simulink model "Verification_simulink_restored_from_autosave"  (R2023a)
settings: Solver=ode15s  StartTime=0.0  StopTime=13  MaxStep=0.001  RelTol=1e-3
values from neighbouring files (symbols this model uses):
  A = [0, 1, 0;K/I, -b_p/I, b_w/I;-K/I, b_p/I, -b_w*I_r]    [LQR.m]    (also in model_verif.m = [0, 1, 0, 0;-K/I, -b_p/I, 0, -b_w/I;0, 0, 0, 1;K/I, b_p/I, 0)
  B = [0;-K_m/I;I_r*K_m]    [LQR.m]    (also in model_verif.m = [0, 0;-K_m/I, 1/I;0, 0;I_r*K_m, -1/I])
  b_p = 0.0314    [CascadePID.m]    (also in LQR.m; model_verif.m = 0.0114)
  b_w = 1/(T*I_r)    (= 0.000346638655462)    [CascadePID.m]    (also in LQR.m; model_verif.m = 0.000315333070556)
  C = tf(num_C,denom_C)    [CascadePID.m]    (also in LQR.m = [1 0 0;0 1 0;0 0 1]; model_verif.m = [1 0 0 0;0 1 0 0;0 0 1 0;0 0 0 1])
  I = 0.011    [CascadePID.m]    (also in LQR.m; model_verif.m = 0.012)
  I_r = (I+I_w)/(I*I_w)    (= 424.242424242)    [CascadePID.m]    (also in LQR.m; model_verif.m = 416.666666667)
  K = 0.597    [CascadePID.m]    (also in Identification_TF.m = X(1); LQR.m; cost_TF.m = ',num2str(K),'; model_verif.m)
  K_m = G*b_w    (= 2.59112394958)    [CascadePID.m]    (also in LQR.m; model_verif.m = 2.3571147024)
  x0 = [20; 0; 0; 0]    [LQR.m]
undefined symbols (not defined in the file or in its folder): DiscIntNeverNeededParam
libraries: slpidlib x3, simulink x1
settings Model: Creator=claraneuburger  LastModifiedBy=claraneuburger

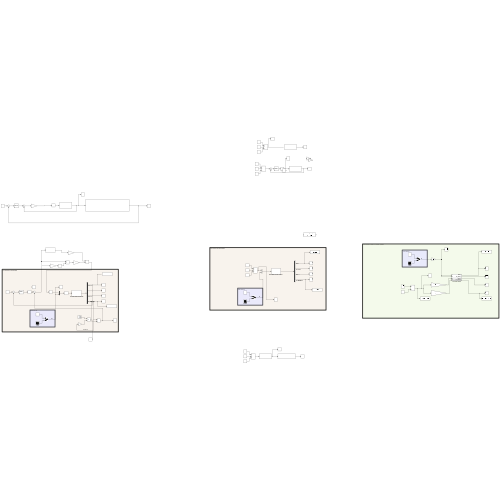
[thumbnail: Simulink's stored preview of the top-level diagram]
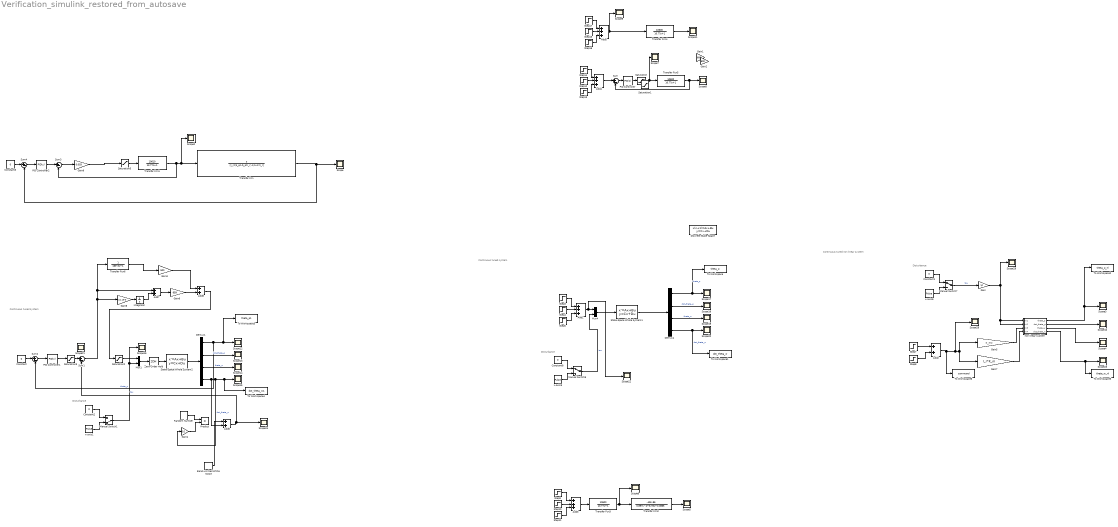
== system Verification_simulink_restored_from_autosave ==
  note: Disturbance
  note: Continuous tuned system
  note: Disturbance
  note: Continuous tuned non linear system
  note: Continuous tuned system
  note: Disturbance
  Add{1,3..5} (4 alike) : Sum  Inputs=+++
  Add{2,6..8} (4 alike) : Sum
  Band-Limited White Noise : simulink/Sources/Band-Limited White Noise  Cov=[0.05]  Ts=0.01  seed=[23341]
  Constant{,1..3,8} (5 alike) : Constant  Value=0
  Demux1 : Demux
  Demux4 : Demux
  Discrete State-Space : DiscreteStateSpace  A=A  B=B  C=C  D=[0,0;0,0;0,0;0,0]  InitialCondition=x0  SampleTime=0.01
  Gain : Gain  Gain=1/I
  Gain1 : Gain  Gain=600
  Gain2 : Gain  Gain=600
  Gain3 : Gain  Gain=500
  Gain4 : Gain  Gain=0.1
  Gain5 : Gain  Gain=K_m/I
  Gain6 : Gain  Gain=659
  Gain7 : Gain  Gain=I_r*K_m
  Gain8 : Gain  Gain=22.1e-3
  Gain9 : Gain  Gain=0.003
  Integrator : Integrator
  Manual Switch1 : ManualSwitch  CurrentSetting=0
  Manual Switch6 : ManualSwitch
  Manual Switch7 : ManualSwitch
  Mux1 : Mux  Inputs=2
  Mux4 : Mux  Inputs=2
  PID Controller : slpidlib/PID Controller  Controller=PID  Form=Parallel  TimeDomain=Continuous-time  UseExternalTs=off  SampleTime=-1  IntegratorMethod=Forward Euler  FilterMethod=Forward Euler  ControllerParametersSource=internal  P=0.002  I=0  UseKiTs=off  D=0  N=0  UseFilter=on  TunerSelectOption=Transfer Function Based (PID Tuner App)  InitialConditionSource=internal  InitialConditionForIntegrator=0  InitialConditionForFilter=0  DifferentiatorICPrevScaledInput=0  ExternalReset=none  TrackingMode=off  Kt=1  LimitOutput=off  SatLimitsSource=internal  UpperSaturationLimit=inf  LowerSaturationLimit=-inf  LinearizeAsGain=on  AntiWindupMode=none  Kb=1  LimitIntegrator=off  UpperIntegratorSaturationLimit=inf  LowerIntegratorSaturationLimit=-inf  POutMin=[]  POutMax=[]  IOutMin=[]  IOutMax=[]  DOutMin=[]  DOutMax=[]  NOutMin=[]  NOutMax=[]  SumOutMin=[]  SumOutMax=[]  SaturationOutMin=[]  SaturationOutMax=[]  PParamMin=[]  PParamMax=[]  IParamMin=[]  IParamMax=[]  DParamMin=[]  DParamMax=[]  NParamMin=[]  NParamMax=[]  KbParamMin=[]  KbParamMax=[]  KtParamMin=[]  KtParamMax=[]  KbOutMin=[]  KbOutMax=[]  KtOutMin=[]  KtOutMax=[]  IntegratorOutMin=[]  IntegratorOutMax=[]  FilterOutMin=[]  FilterOutMax=[]  SumI1OutMin=[]  SumI1OutMax=[]  SumI2OutMin=[]  SumI2OutMax=[]  SumI3OutMin=[]  SumI3OutMax=[]  SumI4OutMin=[]  SumI4OutMax=[]  SumDOutMin=[]  SumDOutMax=[]  DifferentiatorOutMin=[]  DifferentiatorOutMax=[]  FilterDiffOutCoefMin=[]  FilterDiffOutCoefMax=[]  ReciprocalOutMin=[]  ReciprocalOutMax=[]  SumDenOutMin=[]  SumDenOutMax=[]  SumNumOutMin=[]  SumNumOutMax=[]  DivideOutMin=[]  DivideOutMax=[]  UdiffTsProdOutMin=[]  UdiffTsProdOutMax=[]  NTsProdOutMin=[]  NTsProdOutMax=[]  UintegralTsProdOutMin=[]  UintegralTsProdOutMax=[]  UngainTsProdOutMin=[]  UngainTsProdOutMax=[]  ClampingZeroOutDataTypeStr=Inherit: Inherit via back propagation  ClampingZeroOutMin=[]  ClampingZeroOutMax=[]  FilterDenConstantOutDataTypeStr=Inherit: Inherit via back propagation  FilterDenConstantOutMin=[]  FilterDenConstantOutMax=[]  PCopyOutDataTypeStr=Inherit: Inherit via back propagation  PCopyOutMin=[]  PCopyOutMax=[]  NCopyOutDataTypeStr=Inherit: Inherit via back propagation  NCopyOutMin=[]  NCopyOutMax=[]  IntegratorContinuousStateAttributes=''  IntegratorStateMustResolveToSignalObject=off  IntegratorRTWStateStorageClass=Auto  FilterContinuousStateAttributes=''  FilterStateMustResolveToSignalObject=off  FilterRTWStateStorageClass=Auto  ParallelPVariant=InternalParameters  IdealPVariant=Disabled  IVariant=InternalParameters  DVariant=InternalParameters  IntegratorVariant=Continuous  SatVariant=Disabled  AWVariant=Passthrough  PCopyVariant=Disabled  TRVariant=Disabled  FdbkBlocksVariant=Forward  IdealPFdbkVariant=Disabled  SatFdbkVariant=Disabled  DerivativeFilterVariant=ContFilter  NVariant=InternalParameters  NCopyVariant=Disabled  FilterICVariant=InternalICsFilter  IntegratorICVariant=InternalICs  ExternalResetVariant=Disabled  TRSumVariant=Passthrough  SumFdbkVariant=Disabled  SumVariant=Sum_PID  TsampFilterVariant=InternalTs  TsampNgainVariant=Passthrough  TsampIntegralVariant=Disabled_SignalSpec  ExternalSaturationOutDataTypeStr=Inherit: Same as second input
  PID Controller1 : slpidlib/PID Controller  Controller=PID  Form=Parallel  TimeDomain=Discrete-time  UseExternalTs=off  SampleTime=0.01  IntegratorMethod=Forward Euler  FilterMethod=Forward Euler  ControllerParametersSource=internal  P=-3941.34808580242  I=-19558.7721008802  UseKiTs=off  D=-188.491586506074  N=193.809190718502  UseFilter=on  TunerSelectOption=Transfer Function Based (PID Tuner App)  InitialConditionSource=internal  InitialConditionForIntegrator=0  InitialConditionForFilter=0  DifferentiatorICPrevScaledInput=0  ExternalReset=none  TrackingMode=off  Kt=1  LimitOutput=off  SatLimitsSource=internal  UpperSaturationLimit=inf  LowerSaturationLimit=-inf  LinearizeAsGain=on  AntiWindupMode=none  Kb=1  LimitIntegrator=off  UpperIntegratorSaturationLimit=inf  LowerIntegratorSaturationLimit=-inf  POutMin=[]  POutMax=[]  IOutMin=[]  IOutMax=[]  DOutMin=[]  DOutMax=[]  NOutMin=[]  NOutMax=[]  SumOutMin=[]  SumOutMax=[]  SaturationOutMin=[]  SaturationOutMax=[]  PParamMin=[]  PParamMax=[]  IParamMin=[]  IParamMax=[]  DParamMin=[]  DParamMax=[]  NParamMin=[]  NParamMax=[]  KbParamMin=[]  KbParamMax=[]  KtParamMin=[]  KtParamMax=[]  KbOutMin=[]  KbOutMax=[]  KtOutMin=[]  KtOutMax=[]  IntegratorOutMin=[]  IntegratorOutMax=[]  FilterOutMin=[]  FilterOutMax=[]  SumI1OutMin=[]  SumI1OutMax=[]  SumI2OutMin=[]  SumI2OutMax=[]  SumI3OutMin=[]  SumI3OutMax=[]  SumI4OutMin=[]  SumI4OutMax=[]  SumDOutMin=[]  SumDOutMax=[]  DifferentiatorOutMin=[]  DifferentiatorOutMax=[]  FilterDiffOutCoefMin=[]  FilterDiffOutCoefMax=[]  ReciprocalOutMin=[]  ReciprocalOutMax=[]  SumDenOutMin=[]  SumDenOutMax=[]  SumNumOutMin=[]  SumNumOutMax=[]  DivideOutMin=[]  DivideOutMax=[]  UdiffTsProdOutMin=[]  UdiffTsProdOutMax=[]  NTsProdOutMin=[]  NTsProdOutMax=[]  UintegralTsProdOutMin=[]  UintegralTsProdOutMax=[]  UngainTsProdOutMin=[]  UngainTsProdOutMax=[]  ClampingZeroOutDataTypeStr=Inherit: Inherit via back propagation  ClampingZeroOutMin=[]  ClampingZeroOutMax=[]  FilterDenConstantOutDataTypeStr=Inherit: Inherit via back propagation  FilterDenConstantOutMin=[]  FilterDenConstantOutMax=[]  PCopyOutDataTypeStr=Inherit: Inherit via back propagation  PCopyOutMin=[]  PCopyOutMax=[]  NCopyOutDataTypeStr=Inherit: Inherit via back propagation  NCopyOutMin=[]  NCopyOutMax=[]  IntegratorContinuousStateAttributes=''  IntegratorStateMustResolveToSignalObject=off  IntegratorRTWStateStorageClass=Auto  FilterContinuousStateAttributes=''  FilterStateMustResolveToSignalObject=off  FilterRTWStateStorageClass=Auto  ParallelPVariant=InternalParameters  IdealPVariant=Disabled  IVariant=InternalParameters  DVariant=InternalParameters  IntegratorVariant=Discrete  SatVariant=Disabled  AWVariant=Passthrough  PCopyVariant=Disabled  TRVariant=Disabled  FdbkBlocksVariant=Forward  IdealPFdbkVariant=Disabled  SatFdbkVariant=Disabled  DerivativeFilterVariant=ForwardEulerFilter  NVariant=InternalParameters  NCopyVariant=Disabled  FilterICVariant=InternalICsFilter  IntegratorICVariant=InternalICs  ExternalResetVariant=Disabled  TRSumVariant=Passthrough  SumFdbkVariant=Disabled  SumVariant=Sum_PID  TsampFilterVariant=InternalTs  TsampNgainVariant=Passthrough  TsampIntegralVariant=Disabled_SignalSpec  ExternalSaturationOutDataTypeStr=Inherit: Same as second input
  PID Controller2 : slpidlib/PID Controller  Controller=PID  Form=Parallel  TimeDomain=Discrete-time  UseExternalTs=off  SampleTime=0.01  IntegratorMethod=Forward Euler  FilterMethod=Forward Euler  ControllerParametersSource=internal  P=130515.507313953  I=39331.7681676177  UseKiTs=off  D=-1038.52898929221  N=77.1061222235788  UseFilter=on  TunerSelectOption=Transfer Function Based (PID Tuner App)  InitialConditionSource=internal  InitialConditionForIntegrator=0  InitialConditionForFilter=0  DifferentiatorICPrevScaledInput=0  ExternalReset=none  TrackingMode=off  Kt=1  LimitOutput=off  SatLimitsSource=internal  UpperSaturationLimit=inf  LowerSaturationLimit=-inf  LinearizeAsGain=on  AntiWindupMode=none  Kb=1  LimitIntegrator=off  UpperIntegratorSaturationLimit=inf  LowerIntegratorSaturationLimit=-inf  POutMin=[]  POutMax=[]  IOutMin=[]  IOutMax=[]  DOutMin=[]  DOutMax=[]  NOutMin=[]  NOutMax=[]  SumOutMin=[]  SumOutMax=[]  SaturationOutMin=[]  SaturationOutMax=[]  PParamMin=[]  PParamMax=[]  IParamMin=[]  IParamMax=[]  DParamMin=[]  DParamMax=[]  NParamMin=[]  NParamMax=[]  KbParamMin=[]  KbParamMax=[]  KtParamMin=[]  KtParamMax=[]  KbOutMin=[]  KbOutMax=[]  KtOutMin=[]  KtOutMax=[]  IntegratorOutMin=[]  IntegratorOutMax=[]  FilterOutMin=[]  FilterOutMax=[]  SumI1OutMin=[]  SumI1OutMax=[]  SumI2OutMin=[]  SumI2OutMax=[]  SumI3OutMin=[]  SumI3OutMax=[]  SumI4OutMin=[]  SumI4OutMax=[]  SumDOutMin=[]  SumDOutMax=[]  DifferentiatorOutMin=[]  DifferentiatorOutMax=[]  FilterDiffOutCoefMin=[]  FilterDiffOutCoefMax=[]  ReciprocalOutMin=[]  ReciprocalOutMax=[]  SumDenOutMin=[]  SumDenOutMax=[]  SumNumOutMin=[]  SumNumOutMax=[]  DivideOutMin=[]  DivideOutMax=[]  UdiffTsProdOutMin=[]  UdiffTsProdOutMax=[]  NTsProdOutMin=[]  NTsProdOutMax=[]  UintegralTsProdOutMin=[]  UintegralTsProdOutMax=[]  UngainTsProdOutMin=[]  UngainTsProdOutMax=[]  ClampingZeroOutDataTypeStr=Inherit: Inherit via back propagation  ClampingZeroOutMin=[]  ClampingZeroOutMax=[]  FilterDenConstantOutDataTypeStr=Inherit: Inherit via back propagation  FilterDenConstantOutMin=[]  FilterDenConstantOutMax=[]  PCopyOutDataTypeStr=Inherit: Inherit via back propagation  PCopyOutMin=[]  PCopyOutMax=[]  NCopyOutDataTypeStr=Inherit: Inherit via back propagation  NCopyOutMin=[]  NCopyOutMax=[]  IntegratorContinuousStateAttributes=''  IntegratorStateMustResolveToSignalObject=off  IntegratorRTWStateStorageClass=Auto  FilterContinuousStateAttributes=''  FilterStateMustResolveToSignalObject=off  FilterRTWStateStorageClass=Auto  ParallelPVariant=InternalParameters  IdealPVariant=Disabled  IVariant=InternalParameters  DVariant=InternalParameters  IntegratorVariant=Discrete  SatVariant=Disabled  AWVariant=Passthrough  PCopyVariant=Disabled  TRVariant=Disabled  FdbkBlocksVariant=Forward  IdealPFdbkVariant=Disabled  SatFdbkVariant=Disabled  DerivativeFilterVariant=ForwardEulerFilter  NVariant=InternalParameters  NCopyVariant=Disabled  FilterICVariant=InternalICsFilter  IntegratorICVariant=InternalICs  ExternalResetVariant=Disabled  TRSumVariant=Passthrough  SumFdbkVariant=Disabled  SumVariant=Sum_PID  TsampFilterVariant=InternalTs  TsampNgainVariant=Passthrough  TsampIntegralVariant=Disabled_SignalSpec  ExternalSaturationOutDataTypeStr=Inherit: Same as second input
  Product : Product
  Random Number : RandomNumber  SampleTime=0.001
  Saturation{,1..2,5} (4 alike) : Saturate  UpperLimit=2.33  LowerLimit=-2.33
  Saturation3 : Saturate  UpperLimit=10  LowerLimit=-10
  Scope{,2..24,28..29} (26 alike) : Scope
  State-Space Whole System1 : StateSpace  A=A  B=B  C=C  D=[0,0;0,0;0,0;0,0]  InitialCondition=x0
  State-Space Whole System2 : StateSpace  A=A  B=B  C=C  D=[0,0;0,0;0,0;0,0]  InitialCondition=x0
  Step10 : Step  Time=15  After=0.31772  SampleTime=0
  Step11 : Step  Time=19  After=-0.31772  SampleTime=0
  Step12 : Step  Time=15  After=1000  SampleTime=0
  Step13 : Step  Time=19  After=-1000  SampleTime=0
  Step{3,7,9,14,17} (5 alike) : Step  Time=0  After=0  SampleTime=0
  Step15 : Step  Time=15  After=0.31772  SampleTime=0
  Step16 : Step  Time=19  After=-0.31772  SampleTime=0
  Step4 : Step  Time=15  After=0.74  SampleTime=0
  Step5 : Step  Time=16  After=-0.74  SampleTime=0
  Step8 : Step  Before=1  After=0  SampleTime=0
  Sum{,1..4} (5 alike) : Sum  Inputs=|+-
  To Workspace : ToWorkspace  VariableName=theta_p  SaveFormat=Timeseries  SampleTime=-1
  To Workspace1 : ToWorkspace  VariableName=dot_theta_w  SaveFormat=Timeseries  SampleTime=-1
  To Workspace2 : ToWorkspace  VariableName=theta_p_nl  SaveFormat=Timeseries  SampleTime=-1
  To Workspace3 : ToWorkspace  VariableName=theta_p1  SaveFormat=Timeseries  SampleTime=-1
  To Workspace4 : ToWorkspace  VariableName=dot_theta_w1  SaveFormat=Timeseries  SampleTime=-1
  To Workspace5 : ToWorkspace  VariableName=theta_w_nl  SaveFormat=Timeseries  SampleTime=-1
  To Workspace6 : ToWorkspace  VariableName=command  SaveFormat=Timeseries  SampleTime=-1
  Transfer Fcn : TransferFcn  Numerator=[1 0]  Denominator=[I_r/I;b_p/I-b_p*I_r;-K/I+K*I_r]
  Transfer Fcn1 : TransferFcn  Numerator=[10610]  Denominator=[13.77 1]
  Transfer Fcn2 : TransferFcn  Numerator=[-49 -86]  Denominator=[0.897 8.78 0.0865]
  Transfer Fcn3 : TransferFcn  Numerator=[10600]  Denominator=[10.77 1]
  Transfer Fcn4 : TransferFcn  Numerator=[10600]  Denominator=[10.77 1]
  Transfer Fcn5 : TransferFcn  Numerator=[10600]  Denominator=[10.77 1]
  Transfer Fcn6 : TransferFcn  Denominator=[16e-3 1]
  Zero-Order Hold : ZeroOrderHold  SampleTime=0.01
  non linear system : Subsystem
  x-axis1 : DiscretePulseGenerator  PulseType=Time based  Amplitude=2  Period=17  PulseWidth=0.01  PhaseDelay=1
  x-axis5 : DiscretePulseGenerator  PulseType=Time based  Amplitude=2  Period=17  PulseWidth=0.01  PhaseDelay=1
  x-axis6 : DiscretePulseGenerator  PulseType=Time based  Amplitude=2  Period=1  PulseWidth=0.5  PhaseDelay=1
  wires:
  Transfer Fcn1/1 -> Sum3/2, Transfer Fcn/1, Scope2/1
  Transfer Fcn/1 -> Sum4/2, Scope/1
  Demux4/3 -> Scope19/1  "theta_w"
  Demux4/1 -> To Workspace/1, Scope17/1  "theta_p"
  Manual Switch6/1 -> Mux4/2  "tau"
  Demux4/4 -> To Workspace1/1, Scope20/1  "dot_theta_w"
  x-axis5/1 -> Manual Switch6/2
  Demux4/2 -> Scope18/1  "dot_theta_p"
  Constant8/1 -> Manual Switch6/1
  Step5/1 -> Add1/3
  Step4/1 -> Add1/2
  Step3/1 -> Add1/1
  Constant1/1 -> Manual Switch7/1
  Gain5/1 -> non linear system/3(In3)
  Manual Switch7/1 -> Gain/1  "tau"
  x-axis6/1 -> Manual Switch7/2
  Gain7/1 -> non linear system/4(In4)
  non linear system/1(theta_p) -> To Workspace2/1, Scope3/1
  Gain/1 -> Scope29/1, non linear system/2(In2), non linear system/1(In1)
  non linear system/2(dot_theta_p) -> Scope10/1
  non linear system/3(theta_w) -> Scope4/1
  non linear system/4(dot_theta_w) -> To Workspace5/1, Scope23/1
  Add2/1 -> To Workspace6/1, Scope28/1, Gain7/1, Gain5/1
  Step8/1 -> Add2/2
  Mux4/1 -> State-Space Whole System1/1
  State-Space Whole System1/1 -> Demux4/1
  Add1/1 -> Scope22/1, Mux4/1
  Step7/1 -> Add2/1
  Step11/1 -> Add3/3
  Step10/1 -> Add3/2
  Step9/1 -> Add3/1
  Transfer Fcn3/1 -> Scope6/1, Transfer Fcn2/1
  Add3/1 -> Transfer Fcn3/1
  Transfer Fcn2/1 -> Scope5/1
  Step12/1 -> Add4/2
  Transfer Fcn5/1 -> Sum/2, Scope8/1
  Step14/1 -> Add4/1
  Step13/1 -> Add4/3
  Add4/1 -> Sum/1
  Step15/1 -> Add5/2
  Step16/1 -> Add5/3
  Add5/1 -> Transfer Fcn4/1, Scope9/1
  Transfer Fcn4/1 -> Scope11/1
  Step17/1 -> Add5/1
  Sum/1 -> PID Controller/1
  PID Controller/1 -> Saturation/1
  Saturation/1 -> Scope7/1, Transfer Fcn5/1
  State-Space Whole System2/1 -> Demux1/1
  Demux1/3 -> Scope14/1  "theta_w"
  x-axis1/1 -> Manual Switch1/2
  Constant2/1 -> Manual Switch1/1
  Demux1/1 -> To Workspace3/1, Scope12/1, Sum2/2  "theta_p"
  Demux1/4 -> Gain4/1, To Workspace4/1, Scope15/1, Add6/2  "dot_theta_w"
  Manual Switch1/1 -> Scope16/1, Mux1/2  "tau"
  Demux1/2 -> Scope13/1  "dot_theta_p"
  Mux1/1 -> Zero-Order Hold/1
  Saturation2/1 -> Mux1/1
  Sum2/1 -> PID Controller1/1
  Constant/1 -> Sum2/1
  Zero-Order Hold/1 -> State-Space Whole System2/1
  Random Number/1 -> Product/1
  Gain4/1 -> Product/2
  Band-Limited White Noise/1 -> Add6/1
  PID Controller1/1 -> Saturation3/1
  Add6/1 -> Sum1/2, Scope24/1
  Saturation3/1 -> Sum1/1
  Add8/1 -> Saturation2/1
  Sum1/1 -> Gain8/1, Transfer Fcn6/1, Add7/1
  Gain8/1 -> Integrator/1
  Integrator/1 -> Add7/2
  Gain6/1 -> Add8/2
  Add7/1 -> Gain6/1
  Transfer Fcn6/1 -> Gain3/1
  Gain3/1 -> Add8/1
  Sum4/1 -> PID Controller2/1
  Constant3/1 -> Sum4/1
  PID Controller2/1 -> Sum3/1
  Saturation5/1 -> Transfer Fcn1/1
  Sum3/1 -> Gain9/1
  Gain9/1 -> Saturation5/1

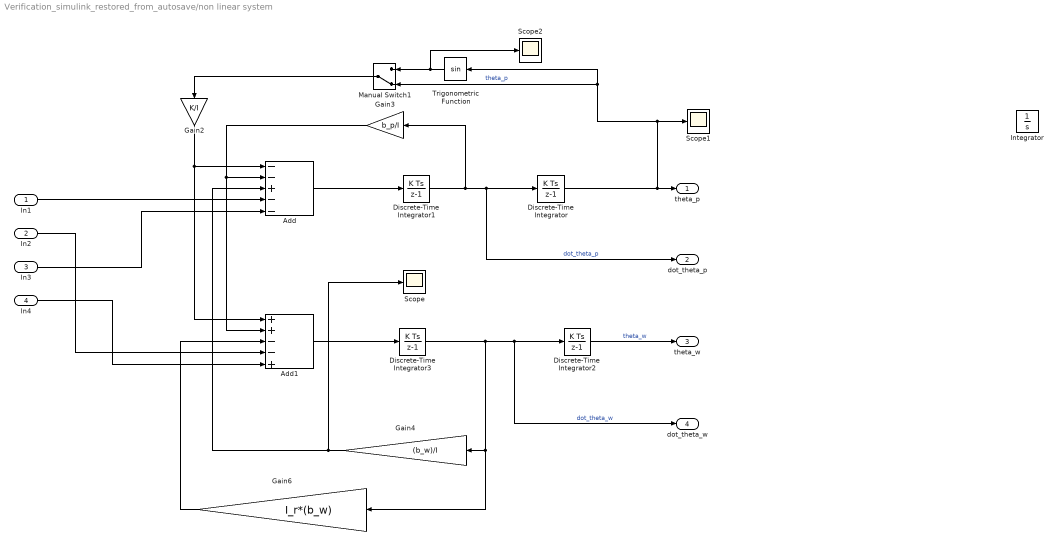
== system Verification_simulink_restored_from_autosave/non linear system ==
  In1 : Inport
  In2 : Inport  Port=2
  In3 : Inport  Port=3
  In4 : Inport  Port=4
  Add : Sum  Inputs=--+--
  Add1 : Sum  Inputs=++--+
  Discrete-Time Integrator{,1..3} (4 alike) : DiscreteIntegrator  SampleTime=0.01  ICPrevOutput=DiscIntNeverNeededParam  ICPrevScaledInput=DiscIntNeverNeededParam
  Gain2 : Gain  Gain=K/I
  Gain3 : Gain  Gain=b_p/I
  Gain4 : Gain  Gain=(b_w)/I
  Gain6 : Gain  Gain=I_r*(b_w)
  Integrator : Integrator
  Manual Switch1 : ManualSwitch  CurrentSetting=0
  Scope : Scope
  Scope1 : Scope
  Scope2 : Scope
  Trigonometric Function : Trigonometry
  theta_p : Outport
  dot_theta_p : Outport  Port=2
  theta_w : Outport  Port=3
  dot_theta_w : Outport  Port=4
  wires:
  In2/1 -> Add1/4
  Trigonometric Function/1 -> Scope2/1, Manual Switch1/1
  In4/1 -> Add1/5
  Gain4/1 -> Scope/1, Add/3
  Gain2/1 -> Add1/1, Add/1
  Gain3/1 -> Add1/2, Add/2
  Discrete-Time Integrator/1 -> Manual Switch1/2, Trigonometric Function/1, Scope1/1, theta_p/1  "theta_p"
  Discrete-Time Integrator1/1 -> dot_theta_p/1, Discrete-Time Integrator/1, Gain3/1  "dot_theta_p"
  Gain6/1 -> Add1/3
  Discrete-Time Integrator3/1 -> Gain6/1, Gain4/1, dot_theta_w/1, Discrete-Time Integrator2/1  "dot_theta_w"
  In1/1 -> Add/4
  Discrete-Time Integrator2/1 -> theta_w/1  "theta_w"
  In3/1 -> Add/5
  Add1/1 -> Discrete-Time Integrator3/1
  Manual Switch1/1 -> Gain2/1
  Add/1 -> Discrete-Time Integrator1/1
